simulink model "MotorXploer"  (R2025b)
settings: Solver=FixedStepAuto  StartTime=0.0  StopTime=20  FixedStep=0.001  RelTol=1e-3  EnableMultiTasking=on
values from neighbouring files (symbols this model uses):
  Time = double(data{4}.Values.Time)    [Lab1_motor_params_student.m]
undefined symbols (not defined in the file or in its folder): Blocking, Continuous, LF, Non
libraries: simulink x5, amg_usbconverter_n_connect_lib x3, eeStairGenerator x2, ctrlSharedLib x1
settings Model: Creator=beamk  LastModifiedBy=ItsMoa
settings OptimizationCC: DefaultParameterBehavior=Inlined  EnhancedBackFolding=on  PassReuseOutputArgsAs=Individual arguments  ZeroExternalMemoryAtStartup=off  ZeroInternalMemoryAtStartup=off  MaxStackSize=64  OptimizeBlockOrder=speed  DifferentSizesBufferReuse=on  OptimizationCustomize=off  EfficientTunableParamExpr=on
settings DebuggingCC: ParameterTunabilityLossMsg=error
settings HardwareCC: ProdBitPerPointer=32.0  ProdBitPerSizeT=32.0  ProdBitPerPtrDiffT=32.0  ProdLargestAtomicInteger=Long  ProdLargestAtomicFloat=Double  ProdWordSize=32.0  ProdLongLongMode=on  ProdHWDeviceType=ARM Compatible->ARM Cortex-M
settings SFSimCC: MATLABDynamicMemAlloc=off
settings RTWCC: SystemTargetFile=ert.tlc  HardwareBoard=STM32G4xx Based  TemplateMakefile=ert_default_tmf  Toolchain=GNU Tools for ARM Embedded Processors  Description=Embedded Coder
settings CodeAppCC: ForceParamTrailComments=on  IgnoreCustomStorageClasses=off  OperatorAnnotations=on  SimulinkDataObjDesc=on  SFDataObjDesc=on  InsertBlockDesc=on
settings ERTTargetCC: ExtModeTransport=3.0  ExtModeStaticAlloc=on  ExtModeStaticAllocSize=2048.0  ExtModeMexFile=ext_xcp  ExtModeIntrfLevel=Level2 - Open  TargetLangStandard=C99 (ISO)  CodeReplacementLibrary=ARM Cortex-M

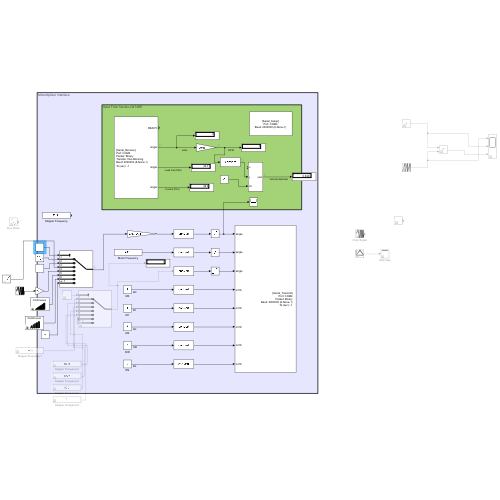
[thumbnail: Simulink's stored preview of the top-level diagram]
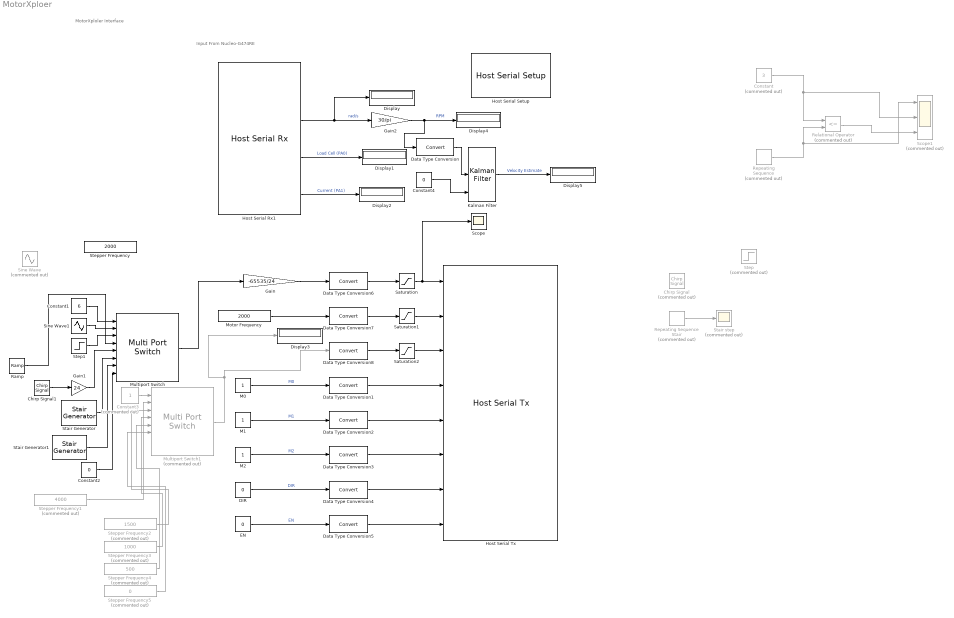
== system MotorXploer ==
  note: Input From Nucleo-G474RE
  note: MotorXploler Interface
  Chirp Signal : simulink/Sources/Chirp Signal  Commented=on  f1=0.1  T=100  f2=1
  Chirp Signal1 : simulink/Sources/Chirp Signal  f1=0  T=10  f2=10
  Constant : Constant  Commented=on  Value=3
  Constant1 : Constant  Value=6  VectorParams1D=off
  Constant2 : Constant  Value=0
  Constant3 : Constant  Commented=on  VectorParams1D=off
  Constant4 : Constant  Value=0
  DIR : Constant  Value=0
  Data Type Conversion{,1..8} (9 alike) : DataTypeConversion  SaturateOnIntegerOverflow=off  RndMeth=Floor
  Display{,1..5} (6 alike) : Display
  EN : Constant  Value=0
  Gain : Gain  Gain=-65535/24
  Gain1 : Gain  Gain=24
  Gain2 : Gain  Gain=30/pi
  Host Serial Rx1 : amg_usbconverter_n_connect_lib/Host Serial Rx  conf=rx  port=<auto>  baudrate=2000000  databits=8  parity=None  stopbit=1  flowcontrol=None  transfer=Non-Blocking  timeout=5  packetmode=Binary  enableinitialvalues=off  initialvalues=[]  binheader='25'  binterminator='4E'  porttype_double=0  porttype_single=3  porttype_int8=0  porttype_uint8=0  porttype_int16=0  porttype_uint16=0  porttype_int32=0  porttype_uint32=0  asciiformat='%f,%f,%d,%d'  rx_asciiterminator="LF (0x0A - \"\\n\")"  tx_asciiterminator="CRLF (0x0D 0x0A - \"\\r\\n\")"  sampletime=-1  enablecustomportlabel=off  cinputportlabel=0  coutputportlabel=A  portpinstr=0  blockid=HostSerialRx1  inputporttype=[]  inputportwidth=[]  inputportlabel={}  outputporttype=[3 1 1 1]  outputportwidth=[1 1 1 1]  outputportlabel={'READY','single','single','single'}  compat=0  optionstring=[]  autoport='COM4'
  Host Serial Setup : amg_usbconverter_n_connect_lib/Host Serial Setup  conf=setup  port=<auto>  baudrate=2000000  databits=8  parity=None  stopbit=1  flowcontrol=None  transfer=Blocking  timeout=2  packetmode=Binary  initialvalues=[]  binheader='7E 7E'  binterminator='03 03'  porttype_double=0  porttype_single=1  porttype_int8=0  porttype_uint8=0  porttype_int16=0  porttype_uint16=0  porttype_int32=0  porttype_uint32=2  asciiformat='%d %u %x'  rx_asciiterminator="CRLF (0x0D 0x0A - \"\\r\\n\")"  tx_asciiterminator="CRLF (0x0D 0x0A - \"\\r\\n\")"  sampletime=-1  enablecustomportlabel=off  cinputportlabel=0  coutputportlabel=A  portpinstr=0  blockid=HostSerialSetup  inputporttype=[]  inputportwidth=[]  inputportlabel={}  outputporttype=[]  outputportwidth=[]  outputportlabel={}  compat=0  optionstring=[]  autoport='COM4'
  Host Serial Tx : amg_usbconverter_n_connect_lib/Host Serial Tx  conf=tx  port=<auto>  baudrate=2000000  databits=8  parity=None  stopbit=1  flowcontrol=None  transfer=Blocking  timeout=2  packetmode=Binary  initialvalues=[]  binheader='25'  binterminator='4E'  porttype_double=0  porttype_single=3  porttype_int8=0  porttype_uint8=0  porttype_int16=5  porttype_uint16=0  porttype_int32=0  porttype_uint32=0  asciiformat='%d,%f'  rx_asciiterminator="CRLF (0x0D 0x0A - \"\\r\\n\")"  tx_asciiterminator="CRLF (0x0D 0x0A - \"\\r\\n\")"  sampletime=-1  enablecustomportlabel=off  cinputportlabel=0  coutputportlabel=A  portpinstr=0  blockid=HostSerialTx  inputporttype=[1 1 1 4 4 4 4 4]  inputportwidth=[1 1 1 1 1 1 1 1]  inputportlabel={'single','single','single','int16','int16','int16','int16','int16'}  outputporttype=[]  outputportwidth=[]  outputportlabel={}  compat=0  optionstring=[]  autoport='COM4'
      settings: SourceProductName=aMG USB Converter N
  Kalman Filter : ctrlSharedLib/Kalman Filter  TimeDomain=Continuous-Time  UseCurrentEstimator=on  ModelSource=LTI State-Space Variable  ModelSourceVariable=ss(0.95,0,1,0)  A=0.95  B=1  C=1  D=0  NumberOfStates=2  NumberOfInputs=0  NumberOfOutputs=1  InitialEstimateSource=Input port  X0=0  P0=10  UseK=off  UseGH=on  NumberOfProcessNoiseInputs=1  G=0  TimeInvariantG=on  H=1  TimeInvariantH=on  Q=1000000  TimeInvariantQ=on  R=0.0001  TimeInvariantR=on  N=0.1  TimeInvariantN=on  AddInputPort=on  AddEnablePort=off  OutputEstimatedY=off  OutputP=off  Ts=-1
  M0 : Constant
  M1 : Constant
  M2 : Constant
  Motor Frequency : Constant  Value=2000  OutDataTypeStr=single
  Multiport Switch : MultiPortSwitch  Inputs=7  SaturateOnIntegerOverflow=off  InputSameDT=off
  Multiport Switch1 : MultiPortSwitch  Commented=on  Inputs=7  SaturateOnIntegerOverflow=off  InputSameDT=off
  Ramp : simulink/Sources/Ramp  slope=5  start=0  InitialOutput=0
  Relational Operator : RelationalOperator  Commented=on  Operator=<=  OutDataTypeStr=boolean  RndMeth=Simplest  InputSameDT=off
  Repeating Sequence : simulink/Sources/Repeating Sequence  Commented=on  rep_seq_t=[0 3]  rep_seq_y=[0 3]
  Repeating Sequence Stair : simulink/Sources/Repeating Sequence Stair  Commented=on  OutValues=[0 1 2 3 4 5 6 7 8 9 10 11 12 11 10 9 8 7 6 5 4 3 2 1].'  tsamp=0.5  OutMin=[]  OutMax=[]  OutDataTypeStr=double  OutputDataTypeScalingMode=double  OutDataType=fixdt(0,8)  ConRadixGroup=Best Precision: Vector-wise  OutScaling=2^-12
  Saturation : Saturate  UpperLimit=65535  LowerLimit=-65535
  Saturation1 : Saturate  UpperLimit=20000  LowerLimit=0
  Saturation2 : Saturate  UpperLimit=inf  LowerLimit=0
  Scope : Scope
      settings: ActiveDisplayYMinimum=-1.4999999999999996  ActiveDisplayYMaximum=13.5
  Scope1 : Scope  Commented=on  NumInputPorts=3
      settings: ActiveDisplayYMinimum=-0.37499999999999989  ActiveDisplayYMaximum=3.375  DataLoggingVariableName=ScopeData2
  Sine Wave : Sin  Commented=on  Amplitude=12  SampleTime=0
  Sine Wave1 : Sin  Amplitude=24  Frequency=pi/2  SampleTime=0
  Stair Generator : eeStairGenerator/Stair Generator  LabelModeActiveChoice=Continuous  TimeInput=[0 2 4 6 8 10 12 14 16 18 20 22 24 26 28 30 32 34 36 38 40 42 44 46 48]  AmplitudeInput=[0 1 0 2 0 3 0 4 0 5 0 6 0 7 0 8 0 9 0 10 0 11 0 12 0]  SampleTime=0  RepeatPattern=off  OutDataTypeStr=double
      settings: LibrarySourceBlock=ee_sl_lib/General Control/Stair Generator
  Stair Generator1 : eeStairGenerator/Stair Generator  LabelModeActiveChoice=Continuous  TimeInput=[0 1.5 3 4.5 6 7.5 9 10.5 12 13.5 15]  AmplitudeInput=[0 8 0 12 0 16 0 20 0 24 0]  SampleTime=0  RepeatPattern=off  OutDataTypeStr=double
      settings: LibrarySourceBlock=ee_sl_lib/General Control/Stair Generator
  Stair step : Scope  Commented=on
      settings: ActiveDisplayYMinimum=-1.3269999999999995  ActiveDisplayYMaximum=21.942999999999998
  Step : Step  Commented=on  After=12  SampleTime=0.1
  Step1 : Step  After=9  SampleTime=0
  Stepper Frequency : Constant  Value=2000  OutDataTypeStr=single
  Stepper Frequency1 : Constant  Commented=on  Value=4000  OutDataTypeStr=single
  Stepper Frequency2 : Constant  Commented=on  Value=1500  OutDataTypeStr=single
  Stepper Frequency3 : Constant  Commented=on  Value=1000  OutDataTypeStr=single
  Stepper Frequency4 : Constant  Commented=on  Value=500  OutDataTypeStr=single
  Stepper Frequency5 : Constant  Commented=on  Value=0  OutDataTypeStr=single
  wires:
  Host Serial Rx1/2 -> Gain2/1, Display/1  "rad/s"
  Host Serial Rx1/3 -> Display1/1  "Load Cell (PA0)"
  M0/1 -> Data Type Conversion1/1  "M0"
  EN/1 -> Data Type Conversion5/1  "EN"
  DIR/1 -> Data Type Conversion4/1  "DIR"
  M1/1 -> Data Type Conversion2/1  "M1"
  M2/1 -> Data Type Conversion3/1  "M2"
  Motor Frequency/1 -> Data Type Conversion7/1
  Data Type Conversion1/1 -> Host Serial Tx/4
  Data Type Conversion2/1 -> Host Serial Tx/5
  Data Type Conversion3/1 -> Host Serial Tx/6
  Data Type Conversion4/1 -> Host Serial Tx/7
  Data Type Conversion5/1 -> Host Serial Tx/8
  Data Type Conversion6/1 -> Saturation/1
  Saturation/1 -> Scope/1, Host Serial Tx/1
  Data Type Conversion7/1 -> Saturation1/1
  Data Type Conversion8/1 -> Saturation2/1
  Saturation1/1 -> Host Serial Tx/2
  Saturation2/1 -> Host Serial Tx/3
  Host Serial Rx1/4 -> Display2/1  "Current (PA1)"
  Gain/1 -> Data Type Conversion6/1
  Repeating Sequence Stair/1 -> Stair step/1
  Repeating Sequence/1 -> Relational Operator/2, Scope1/1
  Constant/1 -> Scope1/2, Relational Operator/1
  Relational Operator/1 -> Scope1/3
  Multiport Switch/1 -> Gain/1
  Constant1/1 -> Multiport Switch/1
  Sine Wave1/1 -> Multiport Switch/2
  Step1/1 -> Multiport Switch/3
  Stair Generator/1 -> Multiport Switch/6
  Stair Generator1/1 -> Multiport Switch/7
  Constant2/1 -> Multiport Switch/8
  Ramp/1 -> Multiport Switch/4
  Chirp Signal1/1 -> Gain1/1
  Gain1/1 -> Multiport Switch/5
  Multiport Switch1/1 -> Display3/1, Data Type Conversion8/1
  Stepper Frequency1/1 -> Multiport Switch1/2
  Stepper Frequency2/1 -> Multiport Switch1/3
  Stepper Frequency3/1 -> Multiport Switch1/4
  Stepper Frequency4/1 -> Multiport Switch1/5
  Stepper Frequency5/1 -> Multiport Switch1/6
  Constant3/1 -> Multiport Switch1/1
  Gain2/1 -> Data Type Conversion/1, Display4/1  "RPM"
  Kalman Filter/1 -> Display5/1  "Velocity Estimate"
  Constant4/1 -> Kalman Filter/3
  Data Type Conversion/1 -> Kalman Filter/2
